simulink model "fuzzycontroller_rfocim"  (R2019a)
settings: Solver=VariableStepAuto  StartTime=0.0  StopTime=10  RelTol=1e-3
settings Model: Creator=ancem  LastModifiedBy=ancem

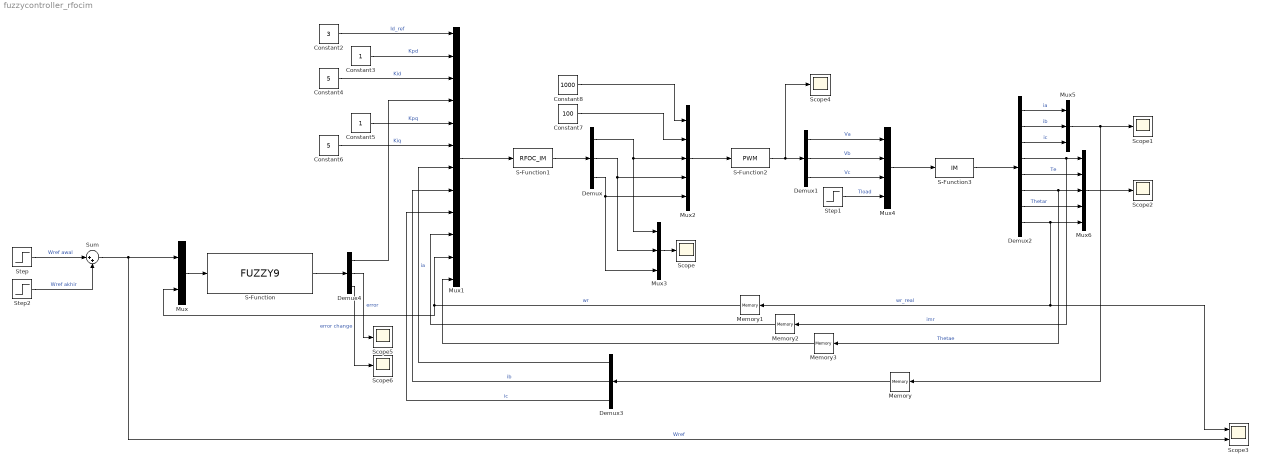
== system fuzzycontroller_rfocim ==
  Constant2 : Constant  Value=3
  Constant3 : Constant
  Constant4 : Constant  Value=5
  Constant5 : Constant
  Constant6 : Constant  Value=5
  Constant7 : Constant  Value=100
  Constant8 : Constant  Value=1000
  Demux{,1,3..4} (4 alike) : Demux  Outputs=3
  Demux2 : Demux  Outputs=8
  Memory{,1..3} (4 alike) : Memory
  Mux : Mux  Inputs=2
  Mux1 : Mux  Inputs=12
  Mux2 : Mux  Inputs=5
  Mux3 : Mux  Inputs=3
  Mux4 : Mux
  Mux5 : Mux  Inputs=3
  Mux6 : Mux  Inputs=5
  S-Function : S-Function  FunctionName=FUZZY9  SFunctionDeploymentMode=off  EnableBusSupport=off
  S-Function1 : S-Function  FunctionName=RFOC_IM  SFunctionDeploymentMode=off  EnableBusSupport=off
  S-Function2 : S-Function  FunctionName=PWM  SFunctionDeploymentMode=off  EnableBusSupport=off
  S-Function3 : S-Function  FunctionName=IM  SFunctionDeploymentMode=off  EnableBusSupport=off
  Scope{,1..2,4..6} (6 alike) : Scope
  Scope3 : Scope  NumInputPorts=2
  Step : Step  After=10  SampleTime=0
  Step1 : Step  Time=3  After=0  SampleTime=0
  Step2 : Step  Time=5  After=-20  SampleTime=0
  Sum : Sum  Inputs=|++
  wires:
  Demux3/1 -> Mux1/7  "ia"
  Demux1/2 -> Mux4/2  "Vb"
  Demux2/8 -> Mux6/5, Scope3/1, Memory1/1  "wr_real"
  Demux2/4 -> Memory2/1, Mux6/1  "imr"
  Mux/1 -> S-Function/1
  Demux3/2 -> Mux1/8  "ib"
  Memory1/1 -> Mux/2, Mux1/11  "wr"
  Demux1/3 -> Mux4/3  "Vc"
  Memory2/1 -> Mux1/10
  Demux/2 -> Mux3/2, Mux2/4
  Demux2/5 -> Mux6/2  "Te"
  S-Function3/1 -> Demux2/1
  Mux3/1 -> Scope/1
  Demux/1 -> Mux2/3, Mux3/1
  Constant2/1 -> Mux1/1  "Id_ref"
  Mux5/1 -> Memory/1, Scope1/1
  Demux2/6 -> Mux6/3, Memory3/1  "Thetae"
  Demux2/3 -> Mux5/3  "ic"
  Constant5/1 -> Mux1/5  "Kpq"
  S-Function2/1 -> Scope4/1, Demux1/1
  Demux2/2 -> Mux5/2  "ib"
  Constant8/1 -> Mux2/1
  Memory3/1 -> Mux1/12
  Step1/1 -> Mux4/4  "Tload"
  Demux2/1 -> Mux5/1  "ia"
  Demux1/1 -> Mux4/1  "Va"
  Mux2/1 -> S-Function2/1
  Demux/3 -> Mux3/3, Mux2/5
  Mux1/1 -> S-Function1/1
  S-Function1/1 -> Demux/1
  Constant6/1 -> Mux1/6  "Kiq"
  Constant4/1 -> Mux1/3  "Kid"
  Mux6/1 -> Scope2/1
  Memory/1 -> Demux3/1
  Constant3/1 -> Mux1/2  "Kpd"
  Constant7/1 -> Mux2/2
  Demux3/3 -> Mux1/9  "ic"
  Demux2/7 -> Mux6/4  "Thetar"
  Mux4/1 -> S-Function3/1
  S-Function/1 -> Demux4/1
  Demux4/1 -> Mux1/4
  Demux4/2 -> Scope5/1  "error"
  Demux4/3 -> Scope6/1  "error change"
  Step/1 -> Sum/1  "Wref awal"
  Sum/1 -> Mux/1, Scope3/2  "Wref"
  Step2/1 -> Sum/2  "Wref akhir"
